simulink model "ANN"  (R2015a)
settings: Solver=ode45  StartTime=0.0  StopTime=10.0  RelTol=1e-3
values from neighbouring files (symbols this model uses):
  alpha = 1    [ANN_params.m]
  anpha_0 = 5    [ANN_params.m]    (also in furuta.m)
  beta0 = 5.8*10^(-4)    (= 0.00058)    [ANN_params.m]    (also in furuta.m)
  beta1 = 1.4142*10^(-3)    (= 0.0014142)    [ANN_params.m]    (also in furuta.m)
  denta1 = 3    [ANN_params.m]
  denta2 = 8    [ANN_params.m]
  g = 9.81    [ANN_params.m]    (also in furuta.m)
  J0 = 4.4*10^(-3)    (= 0.0044)    [ANN_params.m]    (also in furuta.m)
  J1 = 5.5026*10^(-4)    (= 0.00055026)    [ANN_params.m]    (also in furuta.m)
  kd = 0.35    [ANN_params.m]
  kp = 1.05    [ANN_params.m]
  L0 = 0.157    [ANN_params.m]    (also in furuta.m)
  L1 = 0.133    [ANN_params.m]    (also in furuta.m)
  m1 = 0.078    [ANN_params.m]    (also in furuta.m = 0.0933)
  N = 1.05*eye(10)    [ANN_params.m]
  R = 8.53*eye(8)    [ANN_params.m]    (also in furuta.m = [-0.2500,20.6329,-0.6179,2.5406])
  theta_0 = 0    [ANN_params.m]    (also in furuta.m)
  Vhat_0 = zeros(8,10)    [ANN_params.m]
  W0 = [0.5;0.5;0.5;0.5;0.5;0.5;0.5;0.5;0.5;0.5]    [ANN_params.m]
settings Model: Creator=chech  LastModifiedBy=chech

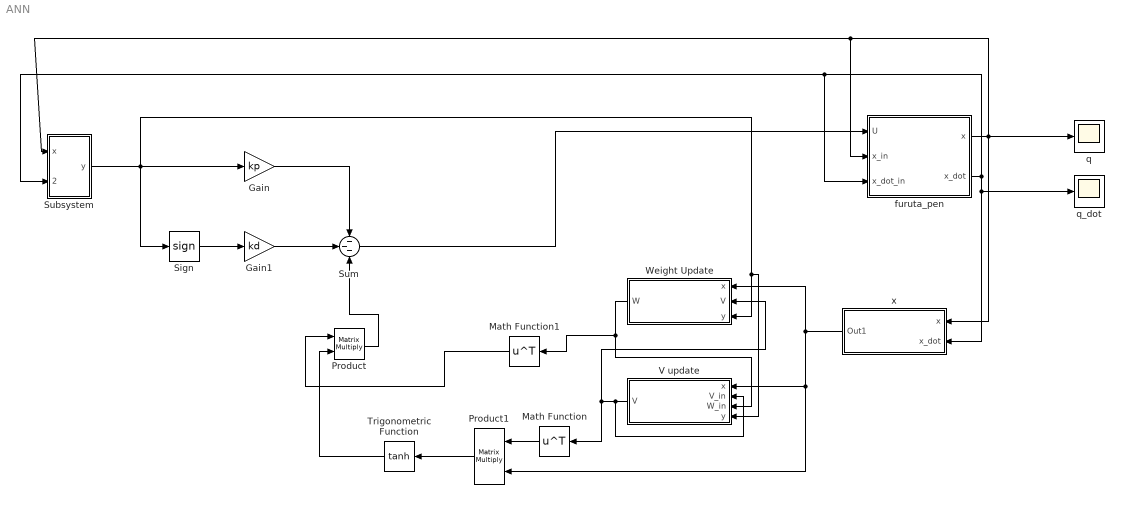
== system ANN ==
  Gain : Gain  Gain=kp
  Gain1 : Gain  Gain=kd
  Math Function : Math  Operator=transpose  SaturateOnIntegerOverflow=on
  Math Function1 : Math  Operator=transpose  SaturateOnIntegerOverflow=on
  Product : Product  Multiplication=Matrix(*)
  Product1 : Product  Multiplication=Matrix(*)
  Sign : Signum
  Subsystem : Subsystem
  Sum : Sum  Inputs=---
  Trigonometric Function : Trigonometry  Operator=tanh
  V update : Subsystem
  Weight Update : Subsystem
  furuta_pen : Subsystem
  q : Scope
      settings: YMin=0  YMax=1750
  q_dot : Scope
  x : Subsystem
  wires:
  furuta_pen/1(x) -> q/1, x/1(x), furuta_pen/2(x_in), Subsystem/1(x)
  furuta_pen/2(x_dot) -> q_dot/1, x/2(x_dot), furuta_pen/3(x_dot_in), Subsystem/2(x_dot)
  Subsystem/1(y) -> Sign/1, V update/4(y), Weight Update/3(y), Gain/1
  Sign/1 -> Gain1/1
  Gain1/1 -> Sum/2
  Gain/1 -> Sum/1
  V update/1(V) -> V update/2(V_in), Math Function/1, Weight Update/2(V)
  Weight Update/1(W) -> Math Function1/1, V update/3(W_in)
  Product/1 -> Sum/3
  Sum/1 -> furuta_pen/1(U)
  Product1/1 -> Trigonometric Function/1
  Trigonometric Function/1 -> Product/2
  Math Function1/1 -> Product/1
  x/1(Out1) -> Product1/2, V update/1(x), Weight Update/1(x)
  Math Function/1 -> Product1/1

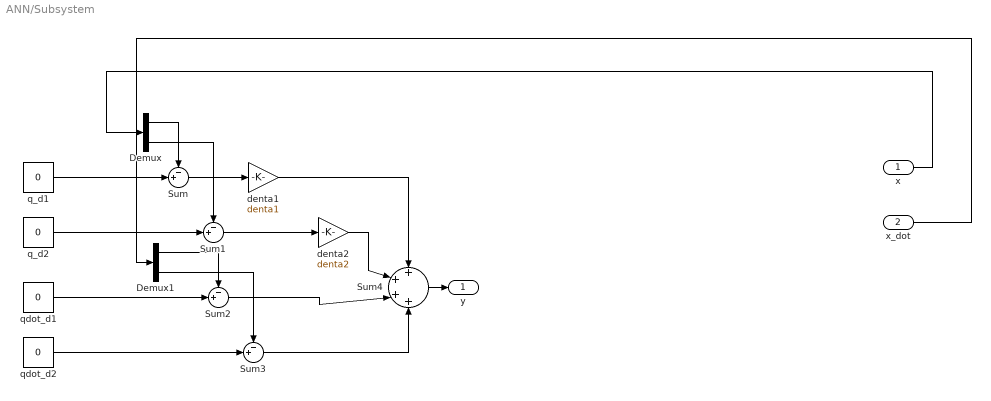
== system ANN/Subsystem ==
  x : Inport
  x_dot : Inport  Port=2
  Demux : Demux  Outputs=2
  Demux1 : Demux  Outputs=2
  Sum{,1..3} (4 alike) : Sum  Inputs=-+|
  Sum4 : Sum  Inputs=++++
  denta1 : Gain  Gain=denta1
  denta2 : Gain  Gain=denta2
  q_d1 : Constant  Value=0
  q_d2 : Constant  Value=0
  qdot_d1 : Constant  Value=0
  qdot_d2 : Constant  Value=0
  y : Outport
  wires:
  Sum2/1 -> Sum4/3
  Sum1/1 -> denta2/1
  Sum3/1 -> Sum4/4
  Sum4/1 -> y/1
  x_dot/1 -> Demux1/1
  Demux/2 -> Sum1/1
  denta1/1 -> Sum4/1
  q_d1/1 -> Sum/2
  q_d2/1 -> Sum1/2
  Demux/1 -> Sum/1
  x/1 -> Demux/1
  Demux1/2 -> Sum3/1
  Demux1/1 -> Sum2/1
  qdot_d1/1 -> Sum2/2
  qdot_d2/1 -> Sum3/2
  Sum/1 -> denta1/1
  denta2/1 -> Sum4/2

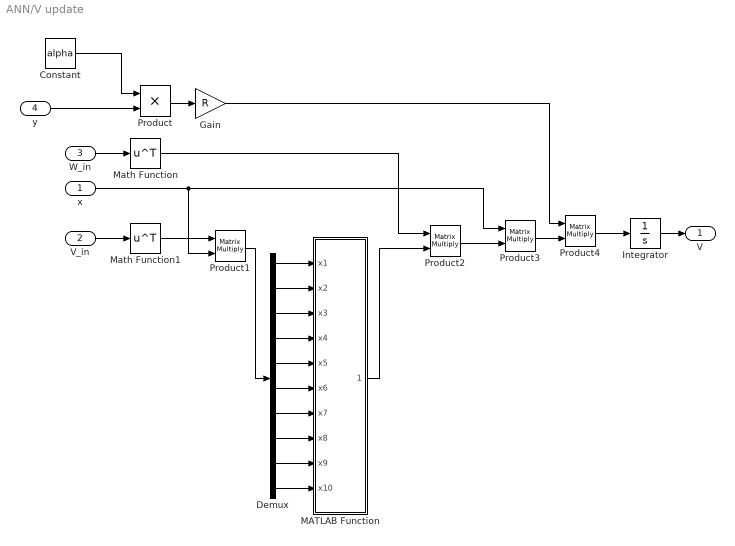
== system ANN/V update ==
  x : Inport
  V_in : Inport  Port=2
  W_in : Inport  Port=3
  y : Inport  Port=4
  Constant : Constant  Value=alpha
  Demux : Demux  Outputs=10
  Gain : Gain  Gain=R
  Integrator : Integrator  InitialCondition=Vhat_0
  MATLAB Function : MATLAB Function  TreatAsAtomicUnit=on
  Math Function : Math  Operator=transpose  SaturateOnIntegerOverflow=on
  Math Function1 : Math  Operator=transpose  SaturateOnIntegerOverflow=on
  Product : Product
  Product{1..4} (4 alike) : Product  Multiplication=Matrix(*)
  V : Outport
  wires:
  y/1 -> Product/2
  Constant/1 -> Product/1
  Product/1 -> Gain/1
  W_in/1 -> Math Function/1
  V_in/1 -> Math Function1/1
  Math Function1/1 -> Product1/1
  x/1 -> Product3/1, Product1/2
  MATLAB Function/1(sigma_dot) -> Product2/2
  Math Function/1 -> Product2/1
  Product2/1 -> Product3/2
  Product3/1 -> Product4/2
  Gain/1 -> Product4/1
  Product4/1 -> Integrator/1
  Integrator/1 -> V/1
  Demux/1 -> MATLAB Function/1(x1)
  Demux/2 -> MATLAB Function/2(x2)
  Demux/3 -> MATLAB Function/3(x3)
  Demux/4 -> MATLAB Function/4(x4)
  Demux/5 -> MATLAB Function/5(x5)
  Demux/6 -> MATLAB Function/6(x6)
  Demux/7 -> MATLAB Function/7(x7)
  Demux/10 -> MATLAB Function/10(x10)
  Demux/9 -> MATLAB Function/9(x9)
  Demux/8 -> MATLAB Function/8(x8)
  Product1/1 -> Demux/1

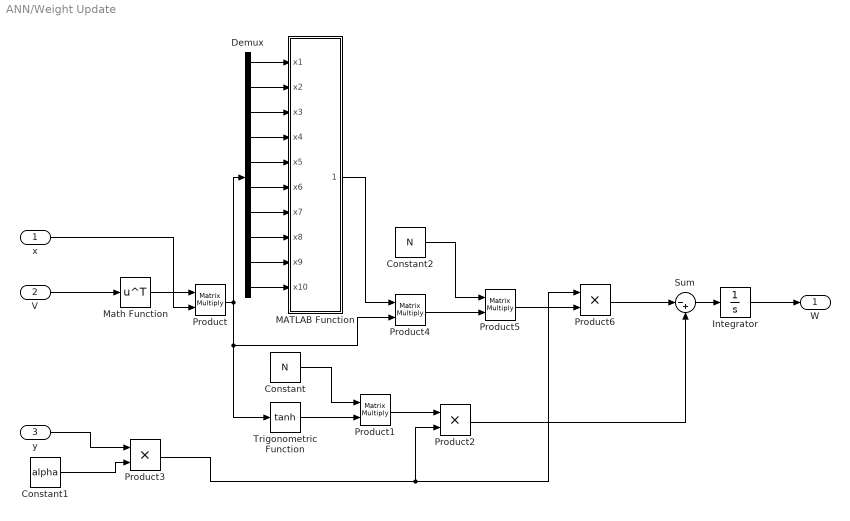
== system ANN/Weight Update ==
  x : Inport
  V : Inport  Port=2
  y : Inport  Port=3
  Constant : Constant  Value=N
  Constant1 : Constant  Value=alpha
  Constant2 : Constant  Value=N
  Demux : Demux  Outputs=10
  Integrator : Integrator  InitialCondition=W0
  MATLAB Function : MATLAB Function  TreatAsAtomicUnit=on
  Math Function : Math  Operator=transpose  SaturateOnIntegerOverflow=on
  Product{,1,4..5} (4 alike) : Product  Multiplication=Matrix(*)
  Product2 : Product
  Product3 : Product
  Product6 : Product
  Sum : Sum  Inputs=|-+
  Trigonometric Function : Trigonometry  Operator=tanh
  W : Outport
  wires:
  V/1 -> Math Function/1
  Math Function/1 -> Product/1
  x/1 -> Product/2
  Trigonometric Function/1 -> Product1/2
  Constant/1 -> Product1/1
  Product1/1 -> Product2/1
  y/1 -> Product3/1
  Constant1/1 -> Product3/2
  Product3/1 -> Product6/1, Product2/2
  Product2/1 -> Sum/2
  MATLAB Function/1(sigma_dot) -> Product4/1
  Product4/1 -> Product5/2
  Constant2/1 -> Product5/1
  Product5/1 -> Product6/2
  Product6/1 -> Sum/1
  Sum/1 -> Integrator/1
  Integrator/1 -> W/1
  Demux/1 -> MATLAB Function/1(x1)
  Demux/2 -> MATLAB Function/2(x2)
  Demux/3 -> MATLAB Function/3(x3)
  Demux/4 -> MATLAB Function/4(x4)
  Demux/5 -> MATLAB Function/5(x5)
  Demux/6 -> MATLAB Function/6(x6)
  Demux/7 -> MATLAB Function/7(x7)
  Product/1 -> Demux/1, Product4/2, Trigonometric Function/1
  Demux/8 -> MATLAB Function/8(x8)
  Demux/9 -> MATLAB Function/9(x9)
  Demux/10 -> MATLAB Function/10(x10)

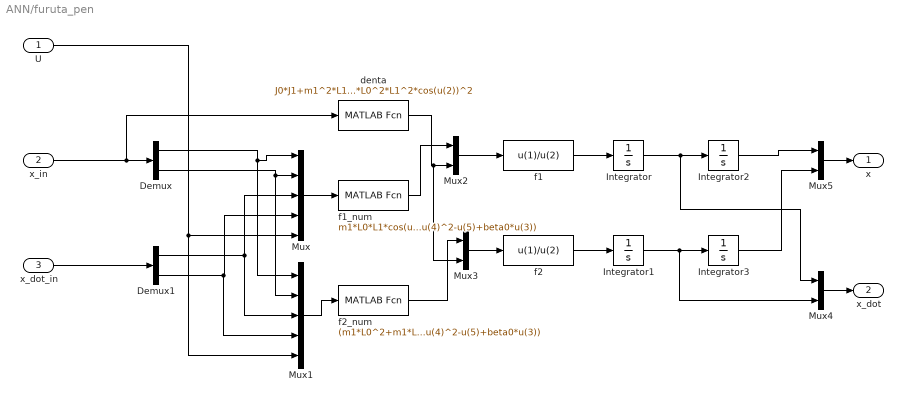
== system ANN/furuta_pen ==
  U : Inport
  x_in : Inport  Port=2
  x_dot_in : Inport  Port=3
  Demux : Demux  Outputs=2
  Demux1 : Demux  Outputs=2
  Integrator : Integrator
  Integrator1 : Integrator
  Integrator2 : Integrator  InitialCondition=theta_0*pi/180
  Integrator3 : Integrator  InitialCondition=anpha_0/180*pi
  Mux : Mux  Inputs=5
  Mux1 : Mux  Inputs=5
  Mux{2..5} (4 alike) : Mux  Inputs=2
  denta : MATLABFcn  MATLABFcn=J0*J1+m1^2*L1^4*sin(u(2))^2+m1^2*L0^2*L1^2+J0*m1*L1^2+J1*m1*L0^2+J1*m1*L1^2*sin(u(2))^2-m1^2*L0^2*L1^2*cos(u(2))^2
  f1 : MATLABFcn  MATLABFcn=u(1)/u(2)
  f1_num : MATLABFcn  MATLABFcn=m1*L0*L1*cos(u(2))*(0.5*m1*L1^2*sin(2*u(2))*u(3)^2+m1*g*L1*sin(u(2))-beta1*u(4))-(m1*L1^2+J1)*(m1*L1^2*sin(2*u(2))*u(3)*u(4)+m1*L0*L1*sin(u(2))*u(4)^2-u(5)+beta0*u(3))
  f2 : MATLABFcn  MATLABFcn=u(1)/u(2)
  f2_num : MATLABFcn  MATLABFcn=(m1*L0^2+m1*L1^2*sin(u(2))^2+J0)*(0.5*m1*L1^2*sin(2*u(2))*u(3)^2+m1*g*L1*sin(u(2))-beta1*u(4))-m1*L0*L1*cos(u(2))*(m1*L1^2*sin(2*u(2))*u(3)*u(4)+m1*L0*L1*sin(u(2))*u(4)^2-u(5)+beta0*u(3))
  x : Outport
  x_dot : Outport  Port=2
  wires:
  x_in/1 -> Demux/1, denta/1
  Mux/1 -> f1_num/1
  Mux1/1 -> f2_num/1
  Mux2/1 -> f1/1
  denta/1 -> Mux3/2, Mux2/2
  f1_num/1 -> Mux2/1
  Mux3/1 -> f2/1
  f2_num/1 -> Mux3/1
  f1/1 -> Integrator/1
  f2/1 -> Integrator1/1
  Integrator/1 -> Mux4/1, Integrator2/1
  Integrator1/1 -> Mux4/2, Integrator3/1
  Mux4/1 -> x_dot/1
  Mux5/1 -> x/1
  Integrator2/1 -> Mux5/1
  Integrator3/1 -> Mux5/2
  U/1 -> Mux1/5, Mux/5
  x_dot_in/1 -> Demux1/1
  Demux/1 -> Mux1/1, Mux/1
  Demux/2 -> Mux1/2, Mux/2
  Demux1/2 -> Mux1/4, Mux/4
  Demux1/1 -> Mux1/3, Mux/3

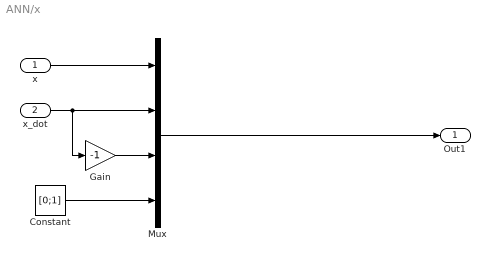
== system ANN/x ==
  x : Inport
  x_dot : Inport  Port=2
  Constant : Constant  Value=[0;1]
  Gain : Gain  Gain=-1
  Mux : Mux
  Out1 : Outport
  wires:
  x/1 -> Mux/1
  x_dot/1 -> Gain/1, Mux/2
  Gain/1 -> Mux/3
  Constant/1 -> Mux/4
  Mux/1 -> Out1/1

== matlab function ANN/Weight Update/MATLAB Function ==
  data: x1 input; sigma_dot output; x2 input; x3 input; x4 input; x5 input; x6 input; x7 input; x8 input; x9 input; x10 input
function sigma_dot = fcn(x1,x2,x3,x4,x5,x6,x7,x8,x9,x10)
%#codegen
%x1=x(1);
%x2=x(2);
%x3=x(3);
%x4=x(4);
%x5=x(5);
%x6=x(6);
%x7=x(7);
%x8=x(8);
%x9=x(9);
%x10=x(10);
sigma_dot = [1-tanh(x1)^2,0,0,0,0,0,0,0,0,0;
    0,1-tanh(x2)^2,0,0,0,0,0,0,0,0;
    0,0,1-tanh(x3)^2,0,0,0,0,0,0,0;
    0,0,0,1-tanh(x4)^2,0,0,0,0,0,0;
    0,0,0,0,1-tanh(x5)^2,0,0,0,0,0;
    0,0,0,0,0,1-tanh(x6)^2,0,0,0,0;
    0,0,0,0,0,0,1-tanh(x7)^2,0,0,0;
    0,0,0,0,0,0,0,1-tanh(x8)^2,0,0;
    0,0,0,0,0,0,0,0,1-tanh(x9)^2,0;
    0,0,0,0,0,0,0,0,0,1-tanh(x10)^2];

== matlab function ANN/V update/MATLAB Function ==
  data: x1 input; sigma_dot output; x2 input; x3 input; x4 input; x5 input; x6 input; x7 input; x8 input; x9 input; x10 input
function sigma_dot = fcn(x1,x2,x3,x4,x5,x6,x7,x8,x9,x10)
%#codegen
%x1=x(1);
%x2=x(2);
%x3=x(3);
%x4=x(4);
%x5=x(5);
%x6=x(6);
%x7=x(7);
%x8=x(8);
%x9=x(9);
%x10=x(10);
sigma_dot = [1-tanh(x1)^2,0,0,0,0,0,0,0,0,0;
    0,1-tanh(x2)^2,0,0,0,0,0,0,0,0;
    0,0,1-tanh(x3)^2,0,0,0,0,0,0,0;
    0,0,0,1-tanh(x4)^2,0,0,0,0,0,0;
    0,0,0,0,1-tanh(x5)^2,0,0,0,0,0;
    0,0,0,0,0,1-tanh(x6)^2,0,0,0,0;
    0,0,0,0,0,0,1-tanh(x7)^2,0,0,0;
    0,0,0,0,0,0,0,1-tanh(x8)^2,0,0;
    0,0,0,0,0,0,0,0,1-tanh(x9)^2,0;
    0,0,0,0,0,0,0,0,0,1-tanh(x10)^2];
